simulink model "Trim_Model_STD"  (R2017b)
settings: configuration reference "cs" (kept outside this file)
values from neighbouring files (symbols this model uses):
  Tr_flap = 0    [TrimFile_STD.m]
undefined symbols (not defined in the file or in its folder): Actuators, Gear
settings Model: Creator=zht  LastModifiedBy=One
settings ConfigSetRef: SourceLocation=Base Workspace

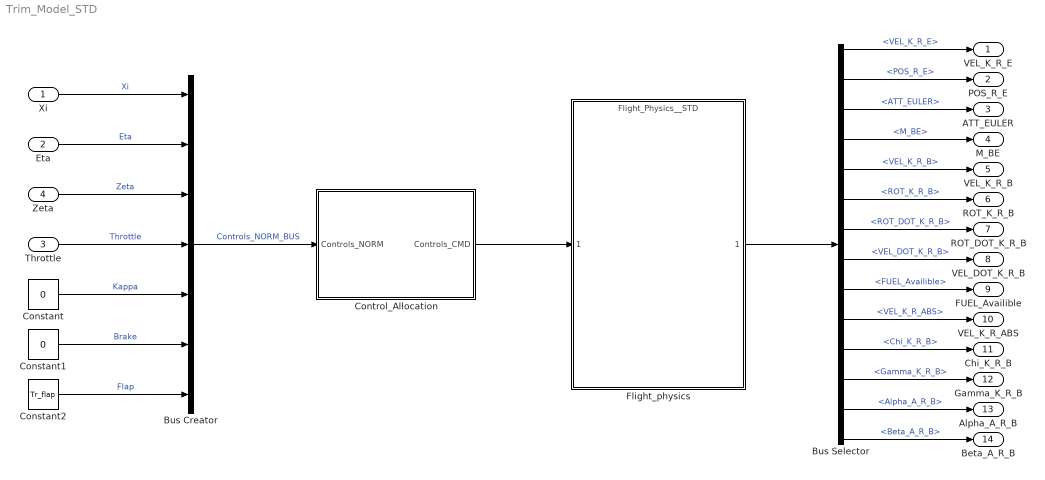
== system Trim_Model_STD ==
  Xi : Inport  OutMin=-1  OutMax=1
  Eta : Inport  Port=2  OutMin=-1  OutMax=1
  Throttle : Inport  Port=3  OutMin=0  OutMax=1
  Zeta : Inport  Port=4  OutMin=-1  OutMax=1
  Bus Creator : BusCreator  Inputs=7
  Bus Selector : BusSelector  OutputSignals=VEL_K_R_E,POS_R_E,ATT_EULER,M_BE,VEL_K_R_B,ROT_K_R_B,ROT_DOT_K_R_B,VEL_DOT_K_R_B,FUEL_Availible,VEL_K_R_ABS,Chi_K_R_B,Gamma_K_R_B,Alpha_A_R_B,Beta_A_R_B
  Constant : Constant  Value=0
  Constant1 : Constant  Value=0
  Constant2 : Constant  Value=Tr_flap
  Control_Allocation : Subsystem
  Flight_physics : ModelReference  ModelNameDialog=Flight_Physics__STD.slx  SimulationMode=Normal  ModelReferenceVersion=1.92
  VEL_K_R_E : Outport
  POS_R_E : Outport  Port=2
  ATT_EULER : Outport  Port=3
  M_BE : Outport  Port=4
  VEL_K_R_B : Outport  Port=5
  ROT_K_R_B : Outport  Port=6
  ROT_DOT_K_R_B : Outport  Port=7
  VEL_DOT_K_R_B : Outport  Port=8
  FUEL_Availible : Outport  Port=9
  VEL_K_R_ABS : Outport  Port=10
  Chi_K_R_B : Outport  Port=11
  Gamma_K_R_B : Outport  Port=12
  Alpha_A_R_B : Outport  Port=13
  Beta_A_R_B : Outport  Port=14
  wires:
  Control_Allocation/1(Controls_CMD) -> Flight_physics/1
  Constant/1 -> Bus Creator/5  "Kappa"
  Bus Creator/1 -> Control_Allocation/1(Controls_NORM)  "Controls_NORM_BUS"
  Zeta/1 -> Bus Creator/3  "Zeta"
  Constant2/1 -> Bus Creator/7  "Flap"
  Throttle/1 -> Bus Creator/4  "Throttle"
  Xi/1 -> Bus Creator/1  "Xi"
  Eta/1 -> Bus Creator/2  "Eta"
  Constant1/1 -> Bus Creator/6  "Brake"
  Flight_physics/1 -> Bus Selector/1
  Bus Selector/1 -> VEL_K_R_E/1  "<VEL_K_R_E>"
  Bus Selector/2 -> POS_R_E/1  "<POS_R_E>"
  Bus Selector/3 -> ATT_EULER/1  "<ATT_EULER>"
  Bus Selector/4 -> M_BE/1  "<M_BE>"
  Bus Selector/5 -> VEL_K_R_B/1  "<VEL_K_R_B>"
  Bus Selector/6 -> ROT_K_R_B/1  "<ROT_K_R_B>"
  Bus Selector/7 -> ROT_DOT_K_R_B/1  "<ROT_DOT_K_R_B>"
  Bus Selector/8 -> VEL_DOT_K_R_B/1  "<VEL_DOT_K_R_B>"
  Bus Selector/9 -> FUEL_Availible/1  "<FUEL_Availible>"
  Bus Selector/10 -> VEL_K_R_ABS/1  "<VEL_K_R_ABS>"
  Bus Selector/11 -> Chi_K_R_B/1  "<Chi_K_R_B>"
  Bus Selector/12 -> Gamma_K_R_B/1  "<Gamma_K_R_B>"
  Bus Selector/13 -> Alpha_A_R_B/1  "<Alpha_A_R_B>"
  Bus Selector/14 -> Beta_A_R_B/1  "<Beta_A_R_B>"

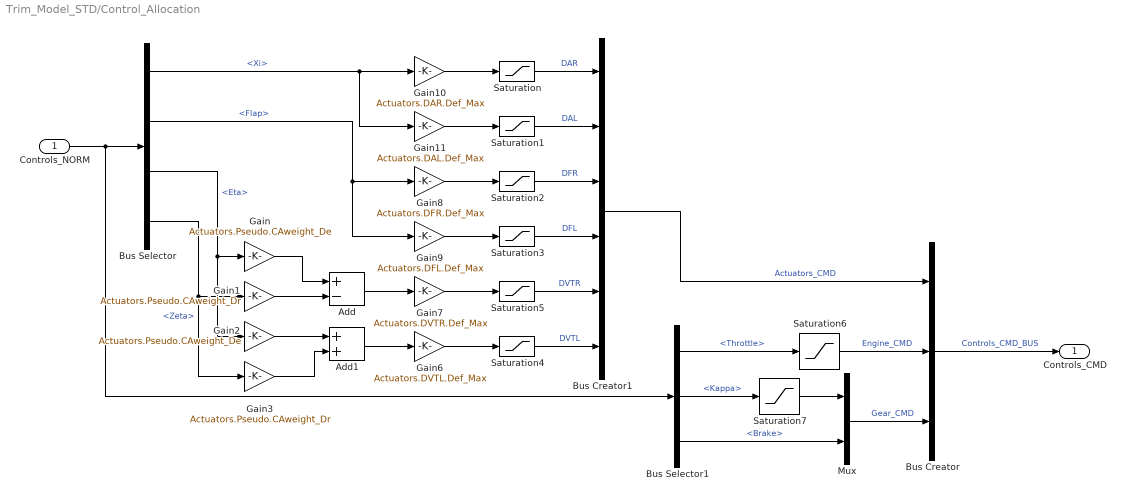
== system Trim_Model_STD/Control_Allocation ==
  Controls_NORM : Inport  OutDataTypeStr=Bus: Controls_NORM_BUS
  Add : Sum  Inputs=+-
  Add1 : Sum
  Bus Creator : BusCreator  Inputs=3  OutDataTypeStr=Bus: Controls_CMD_BUS
  Bus Creator1 : BusCreator  Inputs=6  OutDataTypeStr=Bus: Actuators_CMD_BUS
  Bus Selector : BusSelector  OutputSignals=Xi,Flap,Eta,Zeta
  Bus Selector1 : BusSelector  OutputSignals=Throttle,Kappa,Brake
  Gain : Gain  Gain=Actuators.Pseudo.CAweight_De
  Gain1 : Gain  Gain=Actuators.Pseudo.CAweight_Dr
  Gain10 : Gain  Gain=Actuators.DAR.Def_Max
  Gain11 : Gain  Gain=Actuators.DAL.Def_Max
  Gain2 : Gain  Gain=Actuators.Pseudo.CAweight_De
  Gain3 : Gain  Gain=Actuators.Pseudo.CAweight_Dr
  Gain6 : Gain  Gain=Actuators.DVTL.Def_Max
  Gain7 : Gain  Gain=Actuators.DVTR.Def_Max
  Gain8 : Gain  Gain=Actuators.DFR.Def_Max
  Gain9 : Gain  Gain=Actuators.DFL.Def_Max
  Mux : Mux  Inputs=2
  Saturation : Saturate  UpperLimit=Actuators.DAR.Def_Max  LowerLimit=Actuators.DAR.Def_Min
  Saturation1 : Saturate  UpperLimit=Actuators.DAL.Def_Max  LowerLimit=Actuators.DAL.Def_Min
  Saturation2 : Saturate  UpperLimit=Actuators.DFR.Def_Max  LowerLimit=Actuators.DFR.Def_Min
  Saturation3 : Saturate  UpperLimit=Actuators.DAL.Def_Max  LowerLimit=Actuators.DAL.Def_Min
  Saturation4 : Saturate  UpperLimit=Actuators.DVTL.Def_Max  LowerLimit=Actuators.DVTL.Def_Min
  Saturation5 : Saturate  UpperLimit=Actuators.DVTR.Def_Max  LowerLimit=Actuators.DVTR.Def_Min
  Saturation6 : Saturate  UpperLimit=1  LowerLimit=0
  Saturation7 : Saturate  UpperLimit=Gear.NoseStrut.Def_Max  LowerLimit=-Gear.NoseStrut.Def_Max
  Controls_CMD : Outport  OutDataTypeStr=Bus: Controls_CMD_BUS
  wires:
  Bus Creator/1 -> Controls_CMD/1  "Controls_CMD_BUS"
  Bus Creator1/1 -> Bus Creator/1  "Actuators_CMD"
  Mux/1 -> Bus Creator/3  "Gear_CMD"
  Controls_NORM/1 -> Bus Selector1/1, Bus Selector/1
  Gain2/1 -> Add1/1
  Gain3/1 -> Add1/2
  Gain1/1 -> Add/2
  Gain/1 -> Add/1
  Bus Selector/3 -> Gain2/1, Gain/1  "<Eta>"
  Bus Selector/4 -> Gain3/1, Gain1/1  "<Zeta>"
  Bus Selector/1 -> Gain10/1, Gain11/1  "<Xi>"
  Saturation/1 -> Bus Creator1/1  "DAR"
  Saturation1/1 -> Bus Creator1/2  "DAL"
  Add/1 -> Gain7/1
  Bus Selector/2 -> Gain8/1, Gain9/1  "<Flap>"
  Saturation2/1 -> Bus Creator1/3  "DFR"
  Saturation3/1 -> Bus Creator1/4  "DFL"
  Add1/1 -> Gain6/1
  Bus Selector1/1 -> Saturation6/1  "<Throttle>"
  Saturation5/1 -> Bus Creator1/5  "DVTR"
  Saturation4/1 -> Bus Creator1/6  "DVTL"
  Saturation6/1 -> Bus Creator/2  "Engine_CMD"
  Bus Selector1/2 -> Saturation7/1  "<Kappa>"
  Bus Selector1/3 -> Mux/2  "<Brake>"
  Saturation7/1 -> Mux/1
  Gain6/1 -> Saturation4/1
  Gain7/1 -> Saturation5/1
  Gain8/1 -> Saturation2/1
  Gain9/1 -> Saturation3/1
  Gain10/1 -> Saturation/1
  Gain11/1 -> Saturation1/1
